simulink model "Cheetah_Test"  (R2020b)
settings: Solver=FixedStepAuto  StartTime=0.0  StopTime=10.0  FixedStep=0.001  RelTol=1e-3
values from neighbouring files (symbols this model uses):
  RPY0 = [0; 0; 0]    [Main.m]
  Xs0 = [p0; dp0; omega0; R0(:)]    [Main.m]
undefined symbols (not defined in the file or in its folder): derivedEulerangles, dt_MPC, F_example, fcn1, fcn2, fp_0, fp_example, robotDynamics
settings Model: Creator=Administrator  LastModifiedBy=Administrator

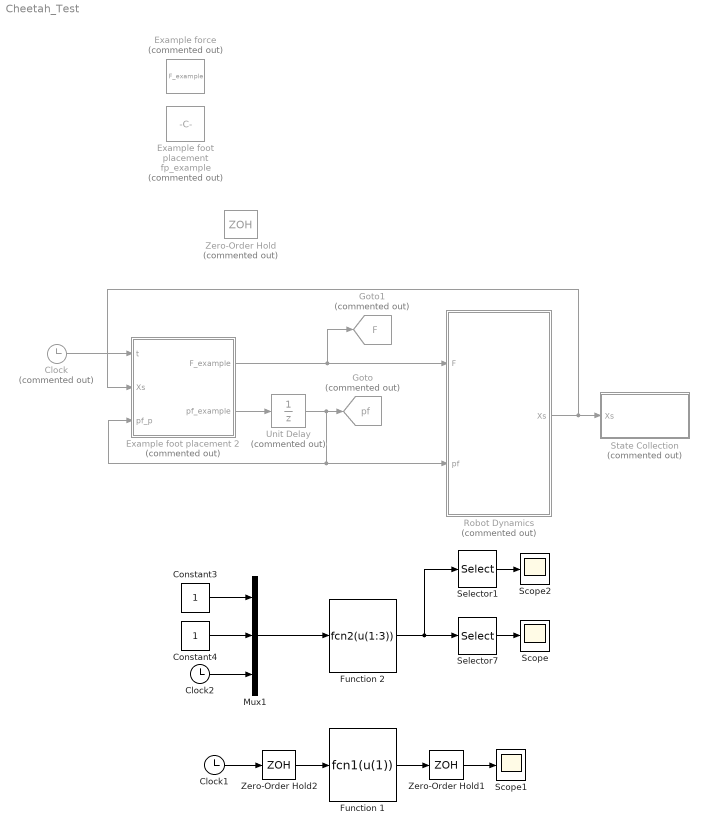
== system Cheetah_Test ==
  Clock : Clock  Commented=on
  Clock1 : Clock
      settings: Decimation=10000
  Clock2 : Clock
      settings: Decimation=10000
  Constant3 : Constant
  Constant4 : Constant
  Example foot placement : Constant  Commented=on  Value=fp_example
  Example foot placement 2 : MATLAB Function  Commented=on  TreatAsAtomicUnit=on
  Example force : Constant  Commented=on  Value=F_example
  Function 1 : MATLABFcn  MATLABFcn=fcn1(u(1))  OutputDimensions=[1 1]  OutputSignalType=real  Output1D=off
  Function 2 : MATLABFcn  MATLABFcn=fcn2(u(1:3))  OutputDimensions=[5 1]  OutputSignalType=real  Output1D=off
  Goto : Goto  Commented=on  GotoTag=pf  TagVisibility=global
  Goto1 : Goto  Commented=on  GotoTag=F  TagVisibility=global
  Mux1 : Mux  Inputs=3
  Robot Dynamics : Subsystem  Commented=on
  Scope : Scope
  Scope1 : Scope
  Scope2 : Scope
  Selector1 : Selector  InputPortWidth=5  IndexOptions=Index vector (dialog)  Indices=[1]  OutputSizes=1
  Selector7 : Selector  InputPortWidth=5  IndexOptions=Index vector (dialog)  Indices=[2:5]  OutputSizes=1
  State Collection : Subsystem  Commented=on
  Unit Delay : UnitDelay  Commented=on  InitialCondition=fp_0  SampleTime=-1  HasFrameUpgradeWarning=on
  Zero-Order Hold : ZeroOrderHold  Commented=on  SampleTime=dt_MPC
  Zero-Order Hold1 : ZeroOrderHold  SampleTime=0.05
  Zero-Order Hold2 : ZeroOrderHold  SampleTime=0.05
  wires:
  Example foot placement 2/2(pf_example) -> Unit Delay/1
  Robot Dynamics/1(Xs) -> Example foot placement 2/2(Xs), State Collection/1(Xs)
  Unit Delay/1 -> Robot Dynamics/2(pf), Example foot placement 2/3(pf_p), Goto/1
  Clock/1 -> Example foot placement 2/1(t)
  Example foot placement 2/1(F_example) -> Robot Dynamics/1(F), Goto1/1
  Constant4/1 -> Mux1/2
  Function 2/1 -> Selector1/1, Selector7/1
  Constant3/1 -> Mux1/1
  Mux1/1 -> Function 2/1
  Selector7/1 -> Scope/1
  Clock2/1 -> Mux1/3
  Function 1/1 -> Zero-Order Hold1/1
  Selector1/1 -> Scope2/1
  Zero-Order Hold1/1 -> Scope1/1
  Clock1/1 -> Zero-Order Hold2/1
  Zero-Order Hold2/1 -> Function 1/1

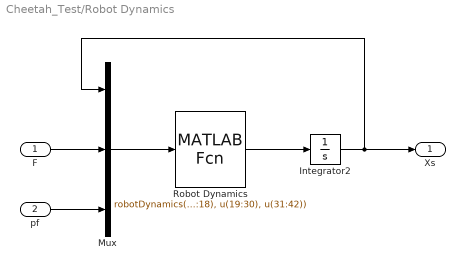
== system Cheetah_Test/Robot Dynamics ==
  F : Inport
  pf : Inport  Port=2
  Integrator2 : Integrator  InitialCondition=Xs0
  Mux : Mux  Inputs=3
  Robot Dynamics : MATLABFcn  MATLABFcn=robotDynamics(u(1:18), u(19:30), u(31:42))  OutputDimensions=[18 1]  OutputSignalType=real  Output1D=off
  Xs : Outport
  wires:
  Mux/1 -> Robot Dynamics/1
  Robot Dynamics/1 -> Integrator2/1
  Integrator2/1 -> Xs/1, Mux/1
  F/1 -> Mux/2
  pf/1 -> Mux/3

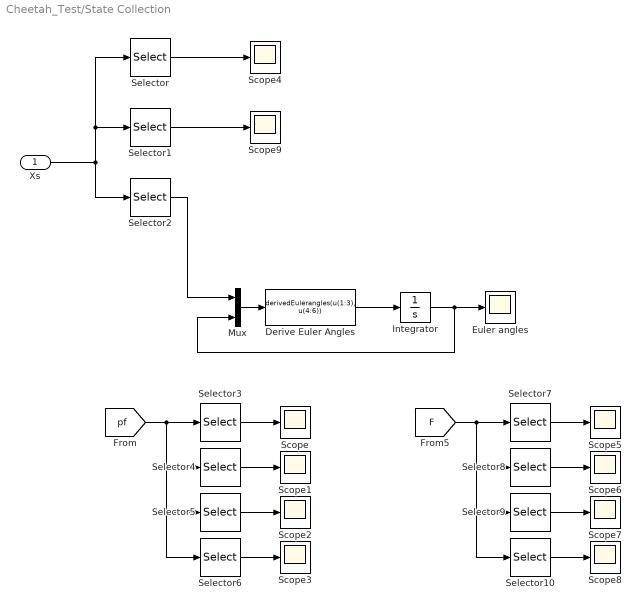
== system Cheetah_Test/State Collection ==
  Xs : Inport
  Derive Euler Angles : MATLABFcn  MATLABFcn=derivedEulerangles(u(1:3), u(4:6))  OutputDimensions=[3 1]  OutputSignalType=real  Output1D=off
  Euler angles : Scope
  Integrator : Integrator  InitialCondition=RPY0
  Mux : Mux  Inputs=2
  Scope{,1..9} (10 alike) : Scope
  Selector : Selector  InputPortWidth=18  IndexOptions=Index vector (dialog)  Indices=[1:3]  OutputSizes=1
  Selector1 : Selector  InputPortWidth=18  IndexOptions=Index vector (dialog)  Indices=[4:6]  OutputSizes=1
  Selector10 : Selector  InputPortWidth=12  IndexOptions=Index vector (dialog)  Indices=[10:12]  OutputSizes=1
  Selector2 : Selector  InputPortWidth=18  IndexOptions=Index vector (dialog)  Indices=[7:9]  OutputSizes=1
  Selector3 : Selector  InputPortWidth=12  IndexOptions=Index vector (dialog)  Indices=[1:3]  OutputSizes=1
  Selector4 : Selector  InputPortWidth=12  IndexOptions=Index vector (dialog)  Indices=[4:6]  OutputSizes=1
  Selector5 : Selector  InputPortWidth=12  IndexOptions=Index vector (dialog)  Indices=[7:9]  OutputSizes=1
  Selector6 : Selector  InputPortWidth=12  IndexOptions=Index vector (dialog)  Indices=[10:12]  OutputSizes=1
  Selector7 : Selector  InputPortWidth=12  IndexOptions=Index vector (dialog)  Indices=[1:3]  OutputSizes=1
  Selector8 : Selector  InputPortWidth=12  IndexOptions=Index vector (dialog)  Indices=[4:6]  OutputSizes=1
  Selector9 : Selector  InputPortWidth=12  IndexOptions=Index vector (dialog)  Indices=[7:9]  OutputSizes=1
  wires:
  Xs/1 -> Selector/1, Selector1/1, Selector2/1
  Selector2/1 -> Mux/1
  Selector1/1 -> Scope9/1
  Selector/1 -> Scope4/1
  Mux/1 -> Derive Euler Angles/1
  Derive Euler Angles/1 -> Integrator/1
  Integrator/1 -> Mux/2, Euler angles/1
  [pf] -> Selector4/1, Selector5/1, Selector6/1, Selector3/1
  Selector3/1 -> Scope/1
  Selector6/1 -> Scope3/1
  Selector5/1 -> Scope2/1
  Selector4/1 -> Scope1/1
  Selector8/1 -> Scope6/1
  Selector9/1 -> Scope7/1
  Selector10/1 -> Scope8/1
  Selector7/1 -> Scope5/1
  [F] -> Selector7/1, Selector10/1, Selector9/1, Selector8/1

== matlab function Cheetah_Test/Example foot placement 2 ==
  data: t input; F_example output size=12; pf_example output; Xs input; pf_p input
function [F_example, pf_example] = fcn(t, Xs, pf_p)
% Trotting gait example

p = Xs(1:3); p_dot = Xs(4:6);
pf_p = reshape(pf_p, [3, 4]);
R = reshape(Xs(10:18), [3, 3]);

l_body = 0.6;
w_body = 0.256;

T_gait = 0.5;
T_stance = T_gait/2;

if mod(floor(t/T_gait), 2) == 0
    % foot 1 and 4 are in contact
    F_example = [R*[43*0.6/2*0; 0; 43*9.8/2]; R*[0; 0; 0]; ...
                  R*[0; 0; 0]; R*[-43*0.6/4*0; 0; 43*9.8/2]];
    
    pf1 = pf_p(:, 1);
    pf2 = p + p_dot*T_stance/2 + R*[ l_body/2;  w_body/2; 0];
    pf3 = p + p_dot*T_stance/2 + R*[-l_body/2; -w_body/2; 0];
    pf4 = pf_p(:, 4);
    pf_example = [pf1; pf2; pf3; pf4];
else
    % foot 2 and 3 are in contact
    F_example = [R*[0; 0; 0]; R*[43*0.6/2*0; 0; 43*9.8/2]; ...
                 R*[-43*0.6/4*0; 0; 43*9.8/2]; R*[0; 0; 0]];
    
    pf1 = p + p_dot*T_stance/2 + R*[ l_body/2; -w_body/2; 0];
    pf2 = pf_p(:, 2);
    pf3 = pf_p(:, 3);
    pf4 = p + p_dot*T_stance/2 + R*[-l_body/2;  w_body/2; 0];
    pf_example = [pf1; pf2; pf3; pf4];
end

end
